simulink model "scdpneumaticlin"  (Simulink 7.6)
settings: Solver=ode23t  StartTime=0.0  StopTime=70  FixedStep=1e-3  MaxStep=1  MinStep=1e-6  RelTol=1e-6
model workspace (MAT data in the model file):
  Ts = 294
  Tc = 294
  Tp = 294
  R = 287
  Ps = 700000
  Pe = 100000
  Vp = 0.000128
  Ws = 0.0045
  Ac = 6.16e-06
  Cs = 0.93
  Cc = 0.909
  Vc = 0.0024
  P0 = 200000
  gam : num (value not decoded)
values from neighbouring files (symbols this model uses):
  gam = 1.403    [scd_aero_guid_dat.m]
  P0 = 101325.0    (= 101325)    [scd_aero_guid_dat.m]
  R = 2    [magballdat.m]    (also in scd_aero_guid_dat.m = 287.26; scdboilerpad.m = diag([1e2,1e6]); scddcmotorpad.m = [2,1.8,2.2])
  Tc = simout.time    [scdcompdelay_engspeed.m]
  Ts = 0.25    [scdcompdelay_engspeed.m]
libraries: scddemolib x4
settings Model: Creator=The MathWorks Inc.
settings SolverCC: ZeroCrossControl=DisableAll
settings DataIOCC: SignalLoggingName=logsOut
settings OptimizationCC: InlineInvariantSignals=on  InitFltsAndDblsToZero=on
settings DebuggingCC: SaveWithParameterizedLinksMsg=none  CheckExecutionContextPreStartOutputMsg=on  CheckExecutionContextRuntimeOutputMsg=on  SignalResolutionControl=TryResolveAllWithWarning  MultiTaskDSMMsg=warning  StrictBusMsg=None
settings SFSimCC: SimParseCustomCode=off
settings GRTTargetCC: TargetFcnLib=ansi_tfl_tmw.mat

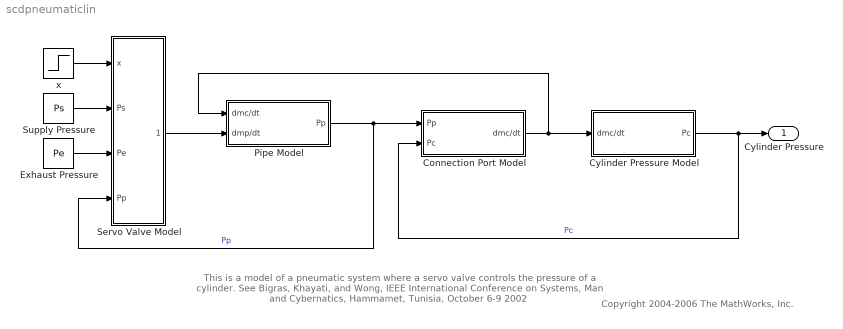
== system scdpneumaticlin ==
  note: This is a model of a pneumatic system where a servo valve controls the pressure of a cylinder.
      | See Bigras, Khayati, and Wong, IEEE International Conference on Systems, Man and Cybernatics, Hammamet, Tunisia, October 6-9 2002
  note: Copyright 2004-2006 The MathWorks, Inc.
  Connection Port Model : Subsystem
  Cylinder Pressure Model : Subsystem
  Exhaust Pressure : Constant  Value=Pe
  Pipe Model : Subsystem
  Servo Valve Model : Subsystem
  Supply Pressure : Constant  Value=Ps
  x : Step  After=0.5e-4  SampleTime=0
  Cylinder Pressure : Outport
  wires:
  Supply Pressure/1 -> Servo Valve Model/2(Ps)
  Exhaust Pressure/1 -> Servo Valve Model/3(Pe)
  Pipe Model/1(Pp) -> Servo Valve Model/4(Pp), Connection Port Model/1(Pp)  "Pp"
  Connection Port Model/1(dmc/dt) -> Cylinder Pressure Model/1(dmc/dt), Pipe Model/1(dmc/dt)
  Cylinder Pressure Model/1(Pc) -> Connection Port Model/2(Pc), Cylinder Pressure/1  "Pc"
  Servo Valve Model/1(dmp/dt) -> Pipe Model/2(dmp/dt)
  x/1 -> Servo Valve Model/1(x)

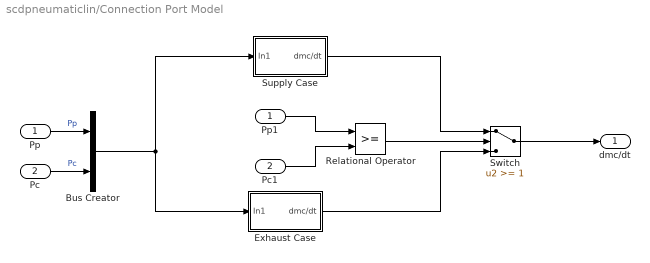
== system scdpneumaticlin/Connection Port Model ==
  Pp : Inport
  Pc : Inport  Port=2
  Bus Creator : BusCreator  Inputs=2
  Exhaust Case : Subsystem
  Pc1 : InportShadow  Port=2
  Pp1 : InportShadow  Port=1
  Relational Operator : RelationalOperator  OutDataTypeStr=boolean
  Supply Case : Subsystem
  Switch : Switch  Threshold=1
  dmc/dt : Outport
  wires:
  Pp/1 -> Bus Creator/1  "Pp"
  Pc/1 -> Bus Creator/2  "Pc"
  Bus Creator/1 -> Exhaust Case/1(In1), Supply Case/1(In1)
  Supply Case/1(dmc/dt) -> Switch/1
  Exhaust Case/1(dmc/dt) -> Switch/3
  Switch/1 -> dmc/dt/1
  Relational Operator/1 -> Switch/2
  Pp1/1 -> Relational Operator/1
  Pc1/1 -> Relational Operator/2

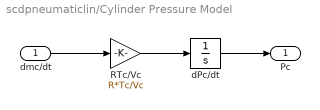
== system scdpneumaticlin/Cylinder Pressure Model ==
  dmc/dt : Inport
  RTc/Vc : Gain  Gain=R*Tc/Vc
  dPc/dt : Integrator  InitialCondition=P0  UpperSaturationLimit=0.7e6  LowerSaturationLimit=0
  Pc : Outport
  wires:
  dPc/dt/1 -> Pc/1
  dmc/dt/1 -> RTc/Vc/1
  RTc/Vc/1 -> dPc/dt/1

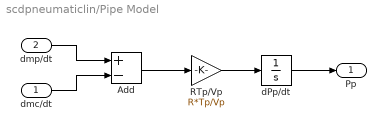
== system scdpneumaticlin/Pipe Model ==
  dmc/dt : Inport
  dmp/dt : Inport  Port=2
  Add : Sum  Inputs=+-
  RTp/Vp : Gain  Gain=R*Tp/Vp
  dPp/dt : Integrator  InitialCondition=P0  UpperSaturationLimit=0.7e6  LowerSaturationLimit=0
  Pp : Outport
  wires:
  RTp/Vp/1 -> dPp/dt/1
  dPp/dt/1 -> Pp/1
  dmp/dt/1 -> Add/1
  dmc/dt/1 -> Add/2
  Add/1 -> RTp/Vp/1

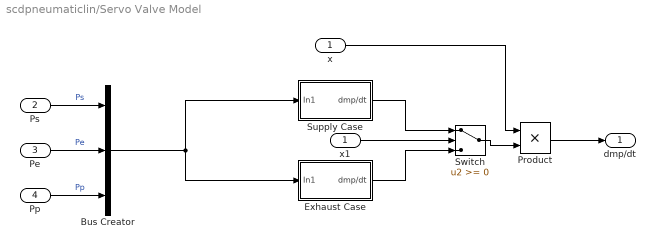
== system scdpneumaticlin/Servo Valve Model ==
  x : Inport
  Ps : Inport  Port=2
  Pe : Inport  Port=3
  Pp : Inport  Port=4
  Bus Creator : BusCreator  Inputs=3
  Exhaust Case : Subsystem
  Product : Product  RndMeth=Zero
  Supply Case : Subsystem
  Switch : Switch
  x1 : InportShadow  Port=1
  dmp/dt : Outport
  wires:
  x/1 -> Product/1
  Ps/1 -> Bus Creator/1  "Ps"
  Pe/1 -> Bus Creator/2  "Pe"
  Pp/1 -> Bus Creator/3  "Pp"
  Bus Creator/1 -> Supply Case/1(In1), Exhaust Case/1(In1)
  Switch/1 -> Product/2
  Product/1 -> dmp/dt/1
  Supply Case/1(dmp/dt) -> Switch/1
  x1/1 -> Switch/2
  Exhaust Case/1(dmp/dt) -> Switch/3

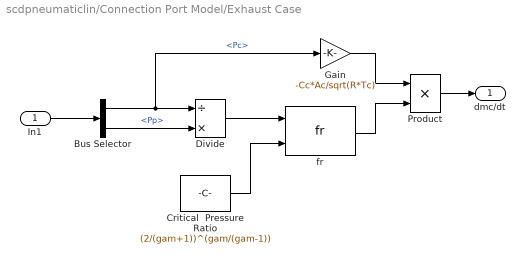
== system scdpneumaticlin/Connection Port Model/Exhaust Case ==
  In1 : Inport
  Bus Selector : BusSelector  OutputSignals=Pc,Pp
  Critical  Pressure Ratio : Constant  Value=(2/(gam+1))^(gam/(gam-1))
  Divide : Product  Inputs=/*
  Gain : Gain  Gain=-Cc*Ac/sqrt(R*Tc)
  Product : Product  Inputs=**
  fr : scddemolib/fr
  dmc/dt : Outport
  wires:
  fr/1 -> Product/2
  Critical  Pressure Ratio/1 -> fr/2
  Divide/1 -> fr/1
  Gain/1 -> Product/1
  Product/1 -> dmc/dt/1
  In1/1 -> Bus Selector/1
  Bus Selector/1 -> Gain/1, Divide/1  "<Pc>"
  Bus Selector/2 -> Divide/2  "<Pp>"

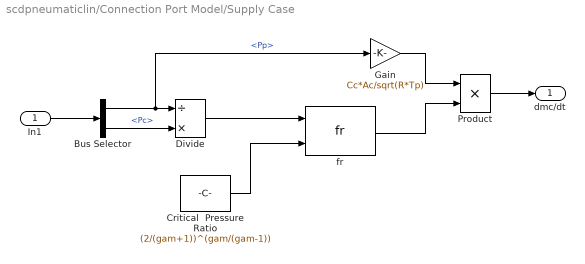
== system scdpneumaticlin/Connection Port Model/Supply Case ==
  In1 : Inport
  Bus Selector : BusSelector  OutputSignals=Pp,Pc
  Critical  Pressure Ratio : Constant  Value=(2/(gam+1))^(gam/(gam-1))
  Divide : Product  Inputs=/*
  Gain : Gain  Gain=Cc*Ac/sqrt(R*Tp)
  Product : Product  Inputs=**
  fr : scddemolib/fr
  dmc/dt : Outport
  wires:
  fr/1 -> Product/2
  Critical  Pressure Ratio/1 -> fr/2
  Divide/1 -> fr/1
  Gain/1 -> Product/1
  Product/1 -> dmc/dt/1
  In1/1 -> Bus Selector/1
  Bus Selector/1 -> Divide/1, Gain/1  "<Pp>"
  Bus Selector/2 -> Divide/2  "<Pc>"

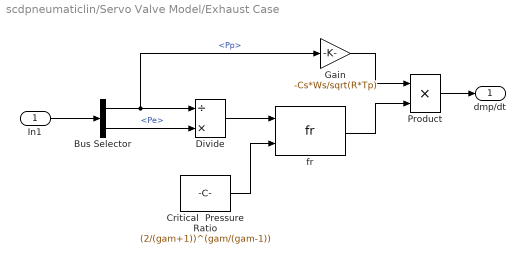
== system scdpneumaticlin/Servo Valve Model/Exhaust Case ==
  In1 : Inport
  Bus Selector : BusSelector  OutputSignals=Pp,Pe
  Critical  Pressure Ratio : Constant  Value=(2/(gam+1))^(gam/(gam-1))
  Divide : Product  Inputs=/*
  Gain : Gain  Gain=-Cs*Ws/sqrt(R*Tp)
  Product : Product  Inputs=**
  fr : scddemolib/fr
  dmp/dt : Outport
  wires:
  In1/1 -> Bus Selector/1
  Bus Selector/1 -> Gain/1, Divide/1  "<Pp>"
  Bus Selector/2 -> Divide/2  "<Pe>"
  Product/1 -> dmp/dt/1
  Gain/1 -> Product/1
  Divide/1 -> fr/1
  Critical  Pressure Ratio/1 -> fr/2
  fr/1 -> Product/2

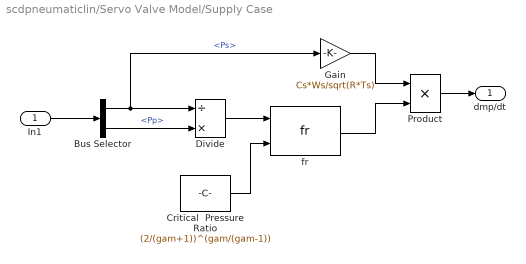
== system scdpneumaticlin/Servo Valve Model/Supply Case ==
  In1 : Inport
  Bus Selector : BusSelector  OutputSignals=Ps,Pp
  Critical  Pressure Ratio : Constant  Value=(2/(gam+1))^(gam/(gam-1))
  Divide : Product  Inputs=/*
  Gain : Gain  Gain=Cs*Ws/sqrt(R*Ts)
  Product : Product  Inputs=**
  fr : scddemolib/fr
  dmp/dt : Outport  InitialOutput=10
  wires:
  In1/1 -> Bus Selector/1
  Product/1 -> dmp/dt/1
  Gain/1 -> Product/1
  Divide/1 -> fr/1
  Critical  Pressure Ratio/1 -> fr/2
  fr/1 -> Product/2
  Bus Selector/2 -> Divide/2  "<Pp>"
  Bus Selector/1 -> Divide/1, Gain/1  "<Ps>"
